simulink model "LowLevelController"  (R2023a)
settings: Solver=VariableStepAuto  StartTime=0.0  StopTime=10.0  RelTol=1e-3
settings Model: Creator=romav  LastModifiedBy=romav

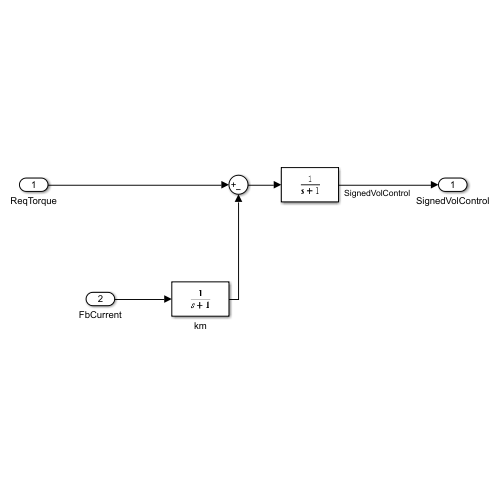
[thumbnail: Simulink's stored preview of the top-level diagram]
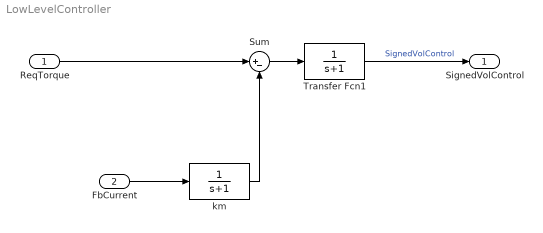
== system LowLevelController ==
  ReqTorque : Inport
  FbCurrent : Inport  Port=2
  Sum : Sum  Inputs=|+-
  Transfer Fcn1 : TransferFcn  Denominator=[1 1]
  km : TransferFcn  Denominator=[1 1]
  SignedVolControl : Outport
  wires:
  FbCurrent/1 -> km/1
  km/1 -> Sum/2
  Transfer Fcn1/1 -> SignedVolControl/1  "SignedVolControl"
  ReqTorque/1 -> Sum/1
  Sum/1 -> Transfer Fcn1/1
